simulink model "QPSK_Transmit_v2"  (R2012b)
settings: Solver=FixedStepDiscrete  StartTime=0.0  StopTime=10  FixedStep=1  RelTol=1e-3
libraries: simulink x21, commutil2 x2
settings Model: Creator=Carl  LastModifiedBy=Christian
settings DataIOCC: SignalLogging=off
settings OptimizationCC: BlockReduction=off  ConditionallyExecuteInputs=off  InlineParams=on
settings DebuggingCC: AlgebraicLoopMsg=error
settings HardwareCC: ProdHWDeviceType=ASIC/FPGA->ASIC/FPGA  ProdEqTarget=off

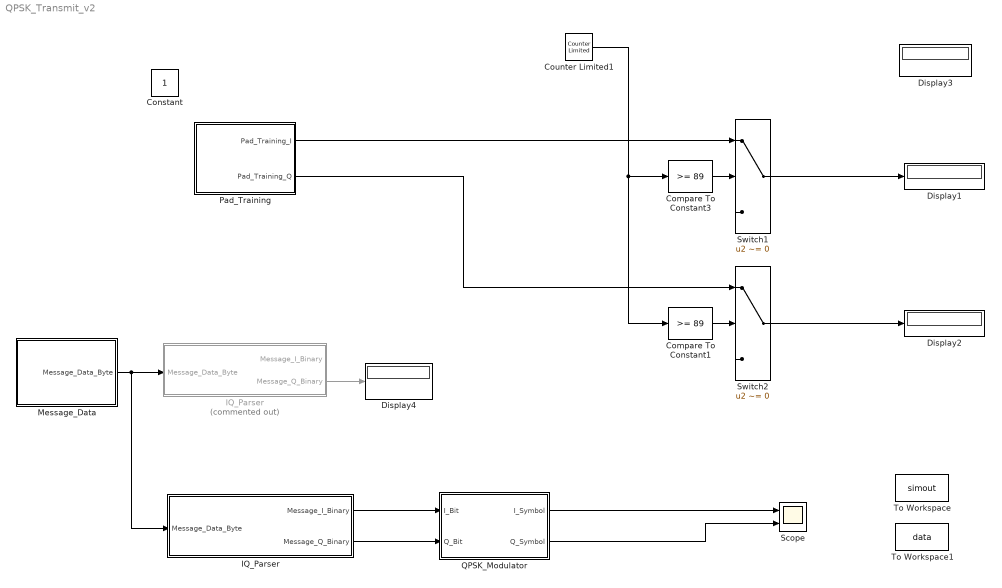
== system QPSK_Transmit_v2 ==
  Compare To Constant1 : simulink/Logic and Bit Operations/Compare To Constant  relop=>=  const=89  OutDataTypeStr=boolean  ZeroCross=off
  Compare To Constant3 : simulink/Logic and Bit Operations/Compare To Constant  relop=>=  const=89  OutDataTypeStr=boolean  ZeroCross=off
  Constant : Constant  OutDataTypeStr=boolean
  Counter Limited1 : simulink/Sources/Counter Limited  uplimit=1023  tsamp=-1
  Display{1..4} (4 alike) : Display
      Display3 settings: Format=binary (Stored Integer)
  IQ_Parser : Subsystem  Commented=on
  "IQ_Parser " : Subsystem
  Message_Data : Subsystem
  Pad_Training : Subsystem
  QPSK_Modulator : Subsystem
  Scope : Scope  NumInputPorts=2
      settings: YMin=-5~-5  YMax=5~5
  Switch1 : Switch  Criteria=u2 ~= 0
  Switch2 : Switch  Criteria=u2 ~= 0
  To Workspace : ToWorkspace  VariableName=simout  SampleTime=-1
  To Workspace1 : ToWorkspace  VariableName=data  SampleTime=-1
  wires:
  Compare To Constant3/1 -> Switch1/2
  Counter Limited1/1 -> Compare To Constant1/1, Compare To Constant3/1
  Switch1/1 -> Display1/1
  Pad_Training/1(Pad_Training_I) -> Switch1/1
  Compare To Constant1/1 -> Switch2/2
  Switch2/1 -> Display2/1
  Pad_Training/2(Pad_Training_Q) -> Switch2/1
  Message_Data/1(Message_Data_Byte) -> "IQ_Parser "/1(Message_Data_Byte), IQ_Parser/1(Message_Data_Byte)
  IQ_Parser/2(Message_Q_Binary) -> Display4/1
  "IQ_Parser "/1(Message_I_Binary) -> QPSK_Modulator/1(I_Bit)
  "IQ_Parser "/2(Message_Q_Binary) -> QPSK_Modulator/2(Q_Bit)
  QPSK_Modulator/1(I_Symbol) -> Scope/1
  QPSK_Modulator/2(Q_Symbol) -> Scope/2

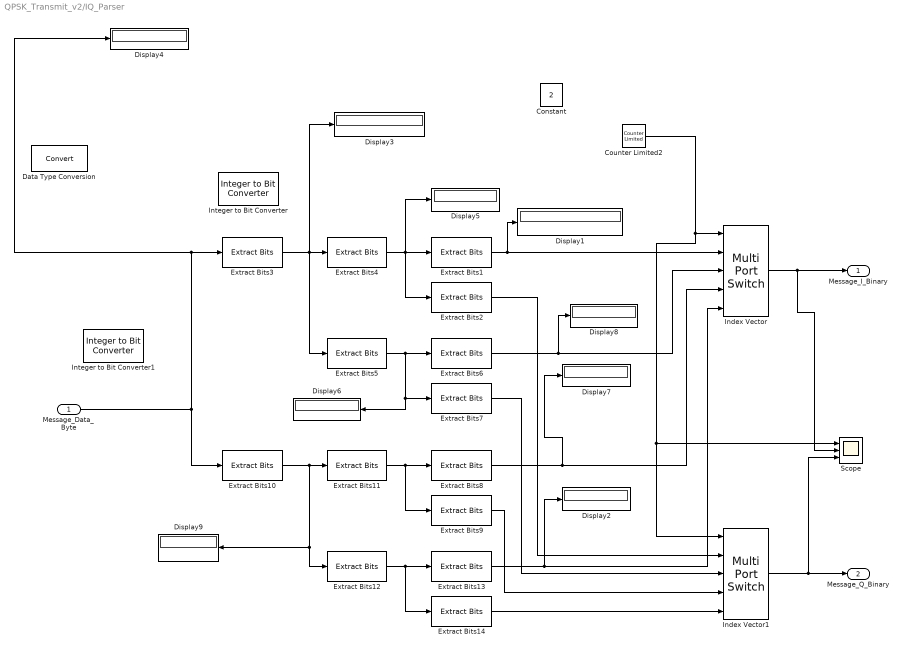
== system QPSK_Transmit_v2/IQ_Parser ==
  Message_Data_Byte : Inport
  Constant : Constant  Value=2
  Counter Limited2 : simulink/Sources/Counter Limited  uplimit=3  tsamp=-1
  Data Type Conversion : DataTypeConversion  ConvertRealWorld=Stored Integer (SI)  RndMeth=Nearest
  Display{1..9} (9 alike) : Display
      Display1 settings: Format=binary (Stored Integer)
      Display3 settings: Format=binary (Stored Integer)
      Display4 settings: Format=binary (Stored Integer)
      Display5 settings: Format=binary (Stored Integer)
      Display6 settings: Format=binary (Stored Integer)
      Display8 settings: Format=binary (Stored Integer)
      Display9 settings: Format=binary (Stored Integer)
  Extract Bits1 : simulink/Logic and Bit Operations/Extract Bits  bitsToExtract=Upper half  numBits=1  bitIdxRange=[15]  outScalingMode=Preserve fixed-point scaling
  Extract Bits10 : simulink/Logic and Bit Operations/Extract Bits  bitsToExtract=Lower half  numBits=2  bitIdxRange=[1 3 5 7]  outScalingMode=Preserve fixed-point scaling
  Extract Bits11 : simulink/Logic and Bit Operations/Extract Bits  bitsToExtract=Upper half  numBits=2  bitIdxRange=[0 2 4 6]  outScalingMode=Preserve fixed-point scaling
  Extract Bits12 : simulink/Logic and Bit Operations/Extract Bits  bitsToExtract=Lower half  numBits=2  bitIdxRange=[0 2 4 6]  outScalingMode=Preserve fixed-point scaling
  Extract Bits13 : simulink/Logic and Bit Operations/Extract Bits  bitsToExtract=Upper half  numBits=1  bitIdxRange=[15]  outScalingMode=Preserve fixed-point scaling
  Extract Bits{2,7,9,14} (4 alike) : simulink/Logic and Bit Operations/Extract Bits  bitsToExtract=Lower half  numBits=1  bitIdxRange=[15]  outScalingMode=Preserve fixed-point scaling
  Extract Bits3 : simulink/Logic and Bit Operations/Extract Bits  bitsToExtract=Upper half  numBits=4  bitIdxRange=[0 2 4 6]  outScalingMode=Preserve fixed-point scaling
  Extract Bits4 : simulink/Logic and Bit Operations/Extract Bits  bitsToExtract=Upper half  numBits=2  bitIdxRange=[0 2 4 6]  outScalingMode=Preserve fixed-point scaling
  Extract Bits5 : simulink/Logic and Bit Operations/Extract Bits  bitsToExtract=Lower half  numBits=2  bitIdxRange=[0 2 4 6]  outScalingMode=Preserve fixed-point scaling
  Extract Bits6 : simulink/Logic and Bit Operations/Extract Bits  bitsToExtract=Range starting with most significant bit  numBits=1  bitIdxRange=[15]  outScalingMode=Preserve fixed-point scaling
  Extract Bits8 : simulink/Logic and Bit Operations/Extract Bits  bitsToExtract=Upper half  numBits=1  bitIdxRange=[15]  outScalingMode=Preserve fixed-point scaling
  Index Vector : MultiPortSwitch  DataPortOrder=Zero-based contiguous  Inputs=4  zeroidx=on
  Index Vector1 : MultiPortSwitch  DataPortOrder=Zero-based contiguous  Inputs=4  zeroidx=on
  Integer to Bit Converter : commutil2/Integer to Bit Converter  nbits=8  signedInputValues=Unsigned  bitOrder=MSB first  outDtype=Inherit via internal rule
  Integer to Bit Converter1 : commutil2/Integer to Bit Converter  nbits=8  signedInputValues=Unsigned  bitOrder=MSB first  outDtype=Inherit via internal rule
  Scope : Scope  NumInputPorts=3
      settings: YMin=-5~-5~-5  YMax=5~5~5
  Message_I_Binary : Outport
  Message_Q_Binary : Outport  Port=2
  wires:
  Index Vector1/1 -> Scope/3, Message_Q_Binary/1
  Extract Bits3/1 -> Display3/1, Extract Bits5/1, Extract Bits4/1
  Extract Bits4/1 -> Display5/1, Extract Bits2/1, Extract Bits1/1
  Extract Bits5/1 -> Extract Bits6/1, Display6/1, Extract Bits7/1
  Extract Bits10/1 -> Extract Bits11/1, Extract Bits12/1, Display9/1
  Extract Bits11/1 -> Extract Bits8/1, Extract Bits9/1
  Extract Bits12/1 -> Extract Bits14/1, Extract Bits13/1
  Extract Bits2/1 -> Index Vector1/2
  Extract Bits7/1 -> Index Vector1/3
  Extract Bits8/1 -> Display7/1, Index Vector/4
  Extract Bits9/1 -> Index Vector1/4
  Extract Bits13/1 -> Display2/1, Index Vector/5
  Extract Bits14/1 -> Index Vector1/5
  Index Vector/1 -> Scope/2, Message_I_Binary/1
  Counter Limited2/1 -> Index Vector1/1, Scope/1, Index Vector/1
  Extract Bits1/1 -> Index Vector/2, Display1/1
  Extract Bits6/1 -> Index Vector/3, Display8/1
  Message_Data_Byte/1 -> Extract Bits10/1, Extract Bits3/1, Display4/1

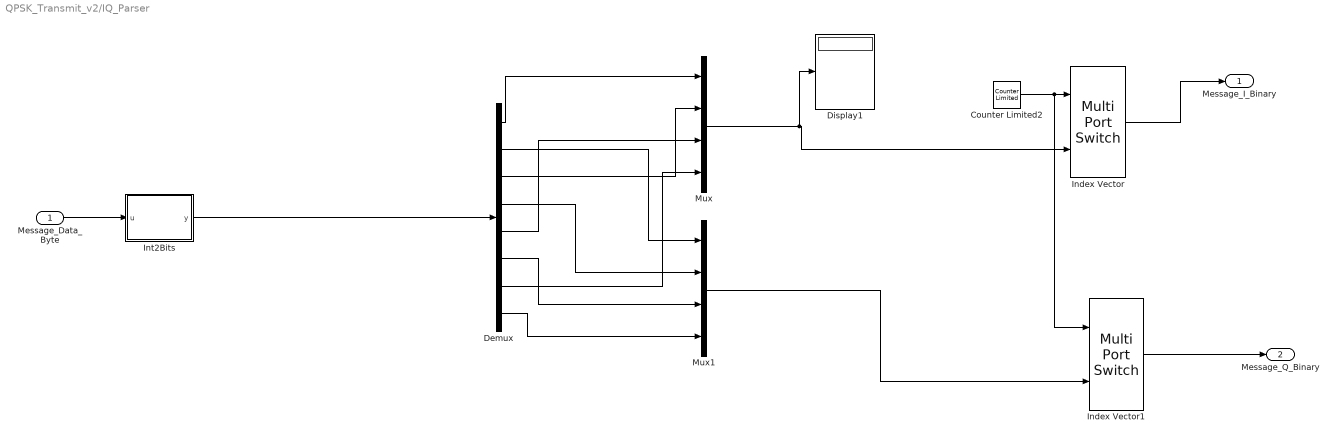
== system QPSK_Transmit_v2/IQ_Parser  ==
  Message_Data_Byte : Inport
  Counter Limited2 : simulink/Sources/Counter Limited  uplimit=3  tsamp=-1
  Demux : Demux  Outputs=8
  Display1 : Display
      settings: Format=binary (Stored Integer)
  Index Vector : MultiPortSwitch  DataPortOrder=Zero-based contiguous  Inputs=1  zeroidx=on
  Index Vector1 : MultiPortSwitch  DataPortOrder=Zero-based contiguous  Inputs=1  zeroidx=on
  Int2Bits : MATLAB Function  TreatAsAtomicUnit=on
  Mux : Mux
  Mux1 : Mux
  Message_I_Binary : Outport
  Message_Q_Binary : Outport  Port=2
  wires:
  Message_Data_Byte/1 -> Int2Bits/1(u)
  Int2Bits/1(y) -> Demux/1
  Demux/1 -> Mux/1
  Demux/2 -> Mux1/1
  Demux/3 -> Mux/2
  Demux/4 -> Mux1/2
  Demux/5 -> Mux/3
  Demux/6 -> Mux1/3
  Demux/7 -> Mux/4
  Demux/8 -> Mux1/4
  Index Vector/1 -> Message_I_Binary/1
  Counter Limited2/1 -> Index Vector1/1, Index Vector/1
  Index Vector1/1 -> Message_Q_Binary/1
  Mux/1 -> Display1/1, Index Vector/2
  Mux1/1 -> Index Vector1/2

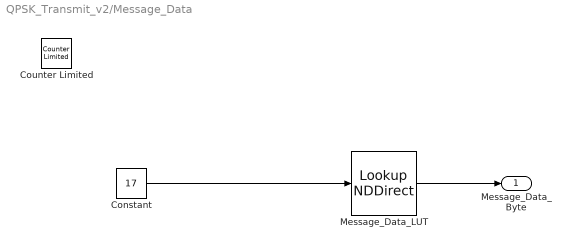
== system QPSK_Transmit_v2/Message_Data ==
  Constant : Constant  Value=17
  Counter Limited : simulink/Sources/Counter Limited  uplimit=17  tsamp=-1
  Message_Data_LUT : LookupNDDirect  NumberOfTableDimensions=1  Table="[12        0        0        1        104        101        108        108        111        32        119        111        114        108        100        33        198        228]"  DiagnosticForOutOfRangeInput=Error  TableDataTypeStr=uint8
  Message_Data_Byte : Outport
  wires:
  Message_Data_LUT/1 -> Message_Data_Byte/1
  Constant/1 -> Message_Data_LUT/1

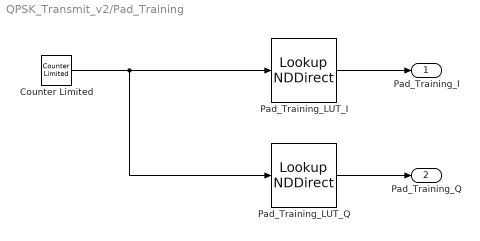
== system QPSK_Transmit_v2/Pad_Training ==
  Counter Limited : simulink/Sources/Counter Limited  uplimit=89  tsamp=-1
  Pad_Training_LUT_I : LookupNDDirect  NumberOfTableDimensions=1  Table=[1,-1,1,-1,1,-1,1,-1,1,-1,1,-1,1,-1,1,-1,1,-1,1,-1,1,-1,1,-1,1,1,1,-1,-1,1,1,-1,-1,1,-1,-1,-1,-1,1,-1,1,1,-1,-1,1,1,1,-1,1,1,1,-1,1,-1,1,1,1,-1,1,1,1,1,-1,1,1,-1,-1,-1,-1,1,1,1,-1,-1,-1,1,1,1,1,-1,1,1,1,1,1,-1,-1,-1,1,1]  DiagnosticForOutOfRangeInput=Error  TableDataTypeStr=int8
  Pad_Training_LUT_Q : LookupNDDirect  NumberOfTableDimensions=1  Table=[1,-1,1,-1,1,-1,1,-1,1,-1,1,-1,1,-1,1,-1,1,-1,1,-1,1,-1,1,-1,1,1,-1,1,1,1,-1,-1,-1,-1,1,1,-1,1,1,-1,-1,-1,1,-1,-1,1,1,1,-1,-1,1,1,1,-1,-1,-1,-1,-1,-1,1,1,-1,1,-1,1,1,-1,-1,1,-1,-1,1,1,-1,-1,-1,-1,-1,1,1,1,1,-1,-1,-1,-1,1,-1,1,-1]  DiagnosticForOutOfRangeInput=Error  TableDataTypeStr=int8
  Pad_Training_I : Outport
  Pad_Training_Q : Outport  Port=2
  wires:
  Pad_Training_LUT_I/1 -> Pad_Training_I/1
  Counter Limited/1 -> Pad_Training_LUT_I/1, Pad_Training_LUT_Q/1
  Pad_Training_LUT_Q/1 -> Pad_Training_Q/1

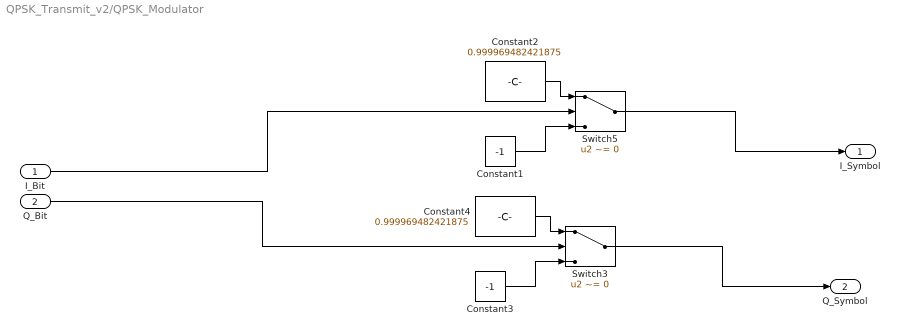
== system QPSK_Transmit_v2/QPSK_Modulator ==
  I_Bit : Inport
  Q_Bit : Inport  Port=2
  Constant1 : Constant  Value=-1  OutDataTypeStr=fixdt(1,16,15)
  Constant2 : Constant  Value=0.999969482421875  OutDataTypeStr=fixdt(1,16,15)
  Constant3 : Constant  Value=-1  OutDataTypeStr=fixdt(1,16,15)
  Constant4 : Constant  Value=0.999969482421875  OutDataTypeStr=fixdt(1,16,15)
  Switch3 : Switch  Criteria=u2 ~= 0  RndMeth=Round
  Switch5 : Switch  Criteria=u2 ~= 0  RndMeth=Round
  I_Symbol : Outport
  Q_Symbol : Outport  Port=2
  wires:
  Constant1/1 -> Switch5/3
  Constant2/1 -> Switch5/1
  I_Bit/1 -> Switch5/2
  Switch5/1 -> I_Symbol/1
  Constant3/1 -> Switch3/3
  Switch3/1 -> Q_Symbol/1
  Constant4/1 -> Switch3/1
  Q_Bit/1 -> Switch3/2

== matlab function QPSK_Transmit_v2/IQ_Parser /Int2Bits ==
  data: u input; y output
function y = fcn(u)
% Converts Integer(8bits) to a 1-D array Bits

y = bitget(u, [8:-1:1])';
